simulink subsystem "Schlitten_Beschleunigung"  (R2020a)
settings: Solver=VariableStepAuto  StartTime=0.0  StopTime=10.0  RelTol=1e-3
undefined symbols (not defined in the file or in its folder): simparams
settings Model: Creator=Tobias  LastModifiedBy=Tobias

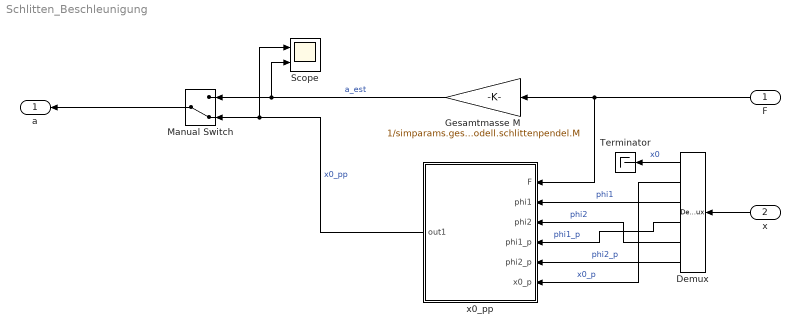
== system Schlitten_Beschleunigung ==
  F : Inport
  x : Inport  Port=2
  Demux : Demux  Outputs=6
  Gesamtmasse M : Gain  Gain=1/simparams.gesamtmodell.schlittenpendel.M
  Manual Switch : ManualSwitch  CurrentSetting=0
  Scope : Scope  NumInputPorts=2
  Terminator : Terminator
  x0_pp : MATLAB Function  TreatAsAtomicUnit=on
  a : Outport
  wires:
  Gesamtmasse M/1 -> Manual Switch/1, Scope/2  "a_est"
  F/1 -> x0_pp/1(F), Gesamtmasse M/1
  Manual Switch/1 -> a/1
  x/1 -> Demux/1
  Demux/1 -> Terminator/1  "x0"
  Demux/2 -> x0_pp/6(x0_p)  "x0_p"
  Demux/3 -> x0_pp/2(phi1)  "phi1"
  Demux/4 -> x0_pp/4(phi1_p)  "phi1_p"
  Demux/5 -> x0_pp/3(phi2)  "phi2"
  Demux/6 -> x0_pp/5(phi2_p)  "phi2_p"
  x0_pp/1(out1) -> Manual Switch/2, Scope/1  "x0_pp"

== matlab function Schlitten_Beschleunigung/x0_pp ==
  data: F input; out1 output; phi1 input; phi2 input; phi1_p input; phi2_p input; x0_p input
function out1 = x0_pp(F,phi1,phi2,phi1_p,phi2_p,x0_p)
%#codegen

%    This function was generated by the Symbolic Math Toolbox version 8.5.
%    27-Aug-2020 12:33:05

t2 = cos(phi1);
t3 = cos(phi2);
t4 = phi1.*2.0;
t5 = phi2.*2.0;
t6 = phi1_p.^2;
t7 = phi2_p.^2;
t8 = -phi2;
t9 = -t5;
t12 = t4+t8;
t10 = phi1+t9;
t13 = t4+t9;
t14 = cos(t12);
t11 = cos(t10);
t15 = cos(t13);
out1 = (F.*(-6.88056773942971e-4)+x0_p.*1.169696515703051e-2-sin(t4).*1.393532095626215e-3+sin(t5).*9.271088396747451e-5+F.*t15.*2.16599243070721e-4+phi1_p.*t2.*2.603497104619667e-5-phi1_p.*t3.*1.251140377267428e-6-phi2_p.*t2.*1.836182779980471e-6+phi2_p.*t3.*1.251140377267428e-6-phi1_p.*t11.*7.299879136949721e-6+phi2_p.*t11.*5.14842607023521e-7+phi1_p.*t14.*1.508756513646403e-6-phi2_p.*t14.*1.508756513646403e-6-t15.*x0_p.*3.682187132202257e-3+t6.*sin(phi1).*7.27408278246111e-5+t7.*sin(phi2).*9.803464946644989e-6+t6.*sin(t10).*2.745414046131636e-6+t7.*sin(t12).*1.408151648240494e-5)./(t15.*3.671558484319389e-3+cos(t4).*1.420522013890127e-4-cos(t5).*9.45065076121045e-6-1.177154833778282e-2);
